simulink library "jud"  (Simulink 8.2)
settings: Solver=ode45  StartTime=0.0  StopTime=10.0  RelTol=1e-3
undefined symbols (not defined in the file or in its folder): ENUM_EPSADASABREASON_GEAR_POSITION_ERROR, ENUM_EPSADASABREASON_THERMAL_ERROR, ENUM_EPSADASABREASON_VEHICLE_SPEED_ERROR, ENUM_EPSLFCSTATUS_NOTAVAIL_PERM, ENUM_EPSLFCSTATUS_NOTAVAIL_TEMP, ENUM_EPSLFCSTATUS_OFF, ENUM_EPSLFCSTATUS_READY, ENUM_EPSLFCSTATUS_TRANSITION, ENUM_EPSLKASTATUS_NOTAVAIL_PERM, ENUM_EPSLKASTATUS_NOTAVAIL_TEMP, ENUM_EPSLKASTATUS_OFF, ENUM_EPSLKASTATUS_READY, ENUM_HMISTATE_ACTIVE, ENUM_KEYSWITCH_ON, ENUM_LFCSTATE_AUTOSTEERING, ENUM_LFCSTATE_STANDBY, ENUM_SENSORSTATE_NORMAL, FALSE, KAPP_VehicleWidth_m, KJUD_EPSLimition_kph, KJUD_EPSLimitionHysis_kph, KJUD_LFC4StandbyDelay_s, KJUD_SoftenTimerThr_s, TRUE, VJUD_LFCOffCount4LKAStandby_s, VJUD_LKAReActingDelay_s, VJUD_TLCTriggerReActingDelay_s
libraries: hcu_lib x12, simulink x10, jcc x1, jcw x1, jeb x1
(part 2 of 3)

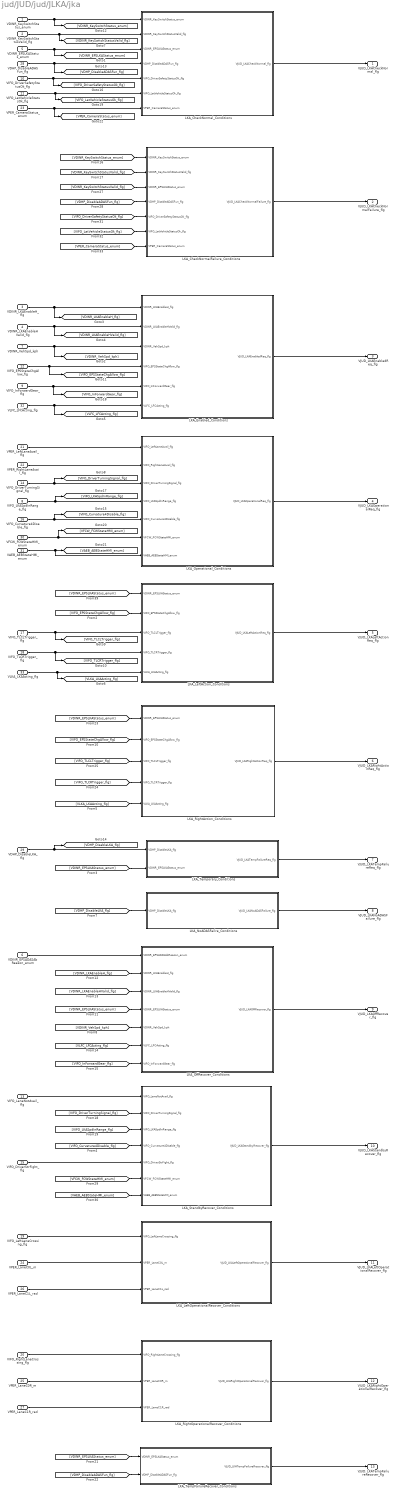
== system jud/JUD/jud/JLKA/jka ==
  VDINR_KeySwitchStatus_enum : Inport
  VDINR_KeySwitchStatusValid_flg : Inport  Port=2
  VDINR_LKAEnableH_flg : Inport  Port=3
  VDINR_LKAEnableHValid_flg : Inport  Port=4
  VDINR_EPSLKAStatus_enum : Inport  Port=5
  VDINR_EPSADASAbReason_enum : Inport  Port=6
  VDINR_VehSpd_kph : Inport  Port=7
  "VIFO_LKASpdInRange_flg " : Inport  Port=8
  VIFO_InForwardGear_flg : Inport  Port=9
  VIFO_DriverSafetyStatusOk_flg : Inport  Port=10
  VIFO_LatVehicleStatusOk_flg : Inport  Port=11
  VIFO_EPSStateChgAllow_flg : Inport  Port=12
  VIFO_LaneNotAvail_flg : Inport  Port=13
  VIFO_DriverTurningSignal_flg : Inport  Port=14
  VIFO_DriverStrFight_flg : Inport  Port=15
  VIFO_Curvature4Disable_flg : Inport  Port=16
  VIFO_TLCLTrigger_flg : Inport  Port=17
  VIFO_TLCRTrigger_flg : Inport  Port=18
  VIFO_LeftLaneCrossing_flg : Inport  Port=19
  VIFO_RightLaneCrossing_flg : Inport  Port=20
  VPER_LeftLaneAvail_flg : Inport  Port=21
  VPER_RightLaneAvail_flg : Inport  Port=22
  VPER_CameraStatus_enum : Inport  Port=23
  VPER_LaneC0L_m : Inport  Port=24
  VPER_LaneC0R_m : Inport  Port=25
  VPER_LaneC1L_rad : Inport  Port=26
  VPER_LaneC1R_rad : Inport  Port=27
  VDHP_DisableADASFun_flg : Inport  Port=28
  VDHP_DisableLKA_flg : Inport  Port=29
  VFCW_FCWStateHMI_enum : Inport  Port=30
  VAEB_AEBStateHMI_enum : Inport  Port=31
  VLFC_LFCActing_flg : Inport  Port=32
  VLKA_LKAActing_flg : Inport  Port=33
  LKA_CheckNormalFailure_Conditions : Subsystem
  LKA_CheckNormal_Conditions : Subsystem
  LKA_Enabled_Conditions : Subsystem
  LKA_LeftAction_Conditions : Subsystem
  LKA_LeftOperationalRecover_Conditions : Subsystem
  LKA_NoADASFailre_Conditions : Subsystem
  LKA_OffRecover_Conditions : Subsystem
  LKA_Operational_Conditions : Subsystem
  LKA_RightAction_Conditions : Subsystem
  LKA_RightOperationalRecover_Conditions : Subsystem
  LKA_StandbyRecover_Conditions : Subsystem
  LKA_TempFailureRecover_Conditions : Subsystem
  LKA_Temporary_Conditions : Subsystem
  VJUD_LKACheckNormal_flg : Outport
  VJUD_LKACheckNormalFailure_flg : Outport  Port=2
  VJUD_LKAEnabledReq_flg : Outport  Port=3
  VJUD_LKAOperationalReq_flg : Outport  Port=4
  VJUD_LKALeftActionReq_flg : Outport  Port=5
  VJUD_LKARightActionReq_flg : Outport  Port=6
  VJUD_LKATempFailureReq_flg : Outport  Port=7
  VJUD_LKANoADASFailure_flg : Outport  Port=8
  VJUD_LKAOffRecover_flg : Outport  Port=9
  VJUD_LKAStandbyRecover_flg : Outport  Port=10
  VJUD_LKALeftOperationalRecover_flg : Outport  Port=11
  VJUD_LKARightOperationalRecover_flg : Outport  Port=12
  VJUD_LKATempFailureRecover_flg : Outport  Port=13
  wires:
  LKA_CheckNormal_Conditions/1(VJUD_LKACheckNormal_flg) -> VJUD_LKACheckNormal_flg/1
  VDINR_KeySwitchStatusValid_flg/1 -> [VDINR_KeySwitchStatusValid_flg], LKA_CheckNormal_Conditions/2(VDINR_KeySwitchStatusValid_flg)
  LKA_Operational_Conditions/1(VJUD_LKAOperationalReq_flg) -> VJUD_LKAOperationalReq_flg/1
  VPER_LeftLaneAvail_flg/1 -> LKA_Operational_Conditions/1(VIFO_LeftLaneAvail_flg)
  VPER_RightLaneAvail_flg/1 -> LKA_Operational_Conditions/2(VIFO_RightLaneAvail_flg)
  VIFO_TLCLTrigger_flg/1 -> [VIFO_TLCLTrigger_flg], LKA_LeftAction_Conditions/3(VIFO_TLCLTrigger_flg)
  LKA_LeftAction_Conditions/1(VJUD_LKALeftActionReq_flg) -> VJUD_LKALeftActionReq_flg/1
  VIFO_DriverSafetyStatusOk_flg/1 -> [VIFO_DriverSafetyStatusOk_flg], LKA_CheckNormal_Conditions/5(VIFO_DriverSafetyStatusOk_flg)
  VDINR_LKAEnableH_flg/1 -> [VDINR_LKAEnableH_flg], LKA_Enabled_Conditions/1(VDINR_LKAEnableH_flg)
  VDINR_LKAEnableHValid_flg/1 -> [VDINR_LKAEnableHValid_flg], LKA_Enabled_Conditions/2(VDINR_LKAEnableHValid_flg)
  LKA_Enabled_Conditions/1(VJUD_LKAEnabledReq_flg) -> VJUD_LKAEnabledReq_flg/1
  VDHP_DisableADASFun_flg/1 -> [VDHP_DisableADASFun_flg], LKA_CheckNormal_Conditions/4(VDHP_DisableADASFun_flg)
  VIFO_EPSStateChgAllow_flg/1 -> [VIFO_EPSStateChgAllow_flg], LKA_Enabled_Conditions/4(VIFO_EPSStateChgAllow_flg)
  VDINR_EPSLKAStatus_enum/1 -> LKA_CheckNormal_Conditions/3(VDINR_EPSLKAStatus_enum), [VDINR_EPSLKAStatus_enum]
  [VDINR_EPSLKAStatus_enum] -> LKA_LeftAction_Conditions/1(VDINR_EPSLKAStatus_enum)
  VIFO_DriverTurningSignal_flg/1 -> [VIFO_DriverTurningSignal_flg], LKA_Operational_Conditions/3(VIFO_DriverTurningSignal_flg)
  VDINR_VehSpd_kph/1 -> [VDINR_VehSpd_kph], LKA_Enabled_Conditions/3(VDINR_VehSpd_kph)
  "VIFO_LKASpdInRange_flg "/1 -> [VIFO_LKASpdInRange_flg], LKA_Operational_Conditions/4(VIFO_LKASpdInRange_flg)
  [VIFO_EPSStateChgAllow_flg] -> LKA_LeftAction_Conditions/2(VIFO_EPSStateChgAllow_flg)
  LKA_Temporary_Conditions/1(VJUD_LKATempFailureReq_flg) -> VJUD_LKATempFailureReq_flg/1
  [VDINR_EPSLKAStatus_enum] -> LKA_Temporary_Conditions/2(VDINR_EPSLKAStatus_enum)
  LKA_NoADASFailre_Conditions/1(VJUD_LKANoADASFailure_flg) -> VJUD_LKANoADASFailure_flg/1
  [VDHP_DisableLKA_flg] -> LKA_NoADASFailre_Conditions/1(VDHP_DisableLKA_flg)
  LKA_OffRecover_Conditions/1(VJUD_LKAOffRecover_flg) -> VJUD_LKAOffRecover_flg/1
  VLFC_LFCActing_flg/1 -> [VLFC_LFCActing_flg], LKA_Enabled_Conditions/6(VLFC_LFCActing_flg)
  [VDINR_VehSpd_kph] -> LKA_OffRecover_Conditions/5(VDINR_VehSpd_kph)
  [VDINR_EPSLKAStatus_enum] -> LKA_OffRecover_Conditions/4(VDINR_EPSLKAStatus_enum)
  VDINR_EPSADASAbReason_enum/1 -> LKA_OffRecover_Conditions/1(VDINR_EPSADASAbReason_enum)
  [VDINR_LKAEnableH_flg] -> LKA_OffRecover_Conditions/2(VDINR_LKAEnableH_flg)
  [VDINR_LKAEnableHValid_flg] -> LKA_OffRecover_Conditions/3(VDINR_LKAEnableHValid_flg)
  [VLFC_LFCActing_flg] -> LKA_OffRecover_Conditions/6(VLFC_LFCActing_flg)
  LKA_StandbyRecover_Conditions/1(VJUD_LKAStandbyRecover_flg) -> VJUD_LKAStandbyRecover_flg/1
  [VIFO_LKASpdInRange_flg] -> LKA_StandbyRecover_Conditions/3(VIFO_LKASpdInRange_flg)
  LKA_LeftOperationalRecover_Conditions/1(VJUD_LKALeftOperationalRecover_flg) -> VJUD_LKALeftOperationalRecover_flg/1
  LKA_TempFailureRecover_Conditions/1(VJUD_LKATempFailureRecover_flg) -> VJUD_LKATempFailureRecover_flg/1
  [VDINR_EPSLKAStatus_enum] -> LKA_TempFailureRecover_Conditions/1(VDINR_EPSLKAStatus_enum)
  [VDHP_DisableADASFun_flg] -> LKA_TempFailureRecover_Conditions/2(VDHP_DisableADASFun_flg)
  VIFO_Curvature4Disable_flg/1 -> [VIFO_Curvature4Disable_flg], LKA_Operational_Conditions/5(VIFO_Curvature4Disable_flg)
  VDHP_DisableLKA_flg/1 -> LKA_Temporary_Conditions/1(VDHP_DisableLKA_flg), [VDHP_DisableLKA_flg]
  [VIFO_Curvature4Disable_flg] -> LKA_StandbyRecover_Conditions/4(VIFO_Curvature4Disable_flg)
  [VIFO_EPSStateChgAllow_flg] -> LKA_RightAction_Conditions/2(VIFO_EPSStateChgAllow_flg)
  [VDINR_EPSLKAStatus_enum] -> LKA_RightAction_Conditions/1(VDINR_EPSLKAStatus_enum)
  LKA_RightAction_Conditions/1(VJUD_LKARightActionReq_flg) -> VJUD_LKARightActionReq_flg/1
  VIFO_TLCRTrigger_flg/1 -> [VIFO_TLCRTrigger_flg], LKA_LeftAction_Conditions/4(VIFO_TLCRTrigger_flg)
  [VIFO_TLCRTrigger_flg] -> LKA_RightAction_Conditions/4(VIFO_TLCRTrigger_flg)
  [VIFO_TLCLTrigger_flg] -> LKA_RightAction_Conditions/3(VIFO_TLCLTrigger_flg)
  VIFO_LatVehicleStatusOk_flg/1 -> [VIFO_LatVehicleStatusOk_flg], LKA_CheckNormal_Conditions/6(VIFO_LatVehicleStatusOk_flg)
  VPER_CameraStatus_enum/1 -> [VPER_CameraStatus_enum], LKA_CheckNormal_Conditions/7(VPER_CameraStatus_enum)
  VIFO_InForwardGear_flg/1 -> LKA_Enabled_Conditions/5(VIFO_InForwardGear_flg), [VIFO_InForwardGear_flg]
  [VIFO_InForwardGear_flg] -> LKA_OffRecover_Conditions/7(VIFO_InForwardGear_flg)
  [VIFO_DriverTurningSignal_flg] -> LKA_StandbyRecover_Conditions/2(VIFO_DriverTurningSignal_flg)
  VIFO_LaneNotAvail_flg/1 -> LKA_StandbyRecover_Conditions/1(VIFO_LaneNotAvail_flg)
  VIFO_DriverStrFight_flg/1 -> LKA_StandbyRecover_Conditions/5(VIFO_DriverStrFight_flg)
  VFCW_FCWStateHMI_enum/1 -> [VFCW_FCWStateHMI_enum], LKA_Operational_Conditions/6(VFCW_FCWStateHMI_enum)
  VAEB_AEBStateHMI_enum/1 -> LKA_Operational_Conditions/7(VAEB_AEBStateHMI_enum), [VAEB_AEBStateHMI_enum]
  LKA_RightOperationalRecover_Conditions/1(VJUD_LKARightOperationalRecover_flg) -> VJUD_LKARightOperationalRecover_flg/1
  VPER_LaneC1L_rad/1 -> LKA_LeftOperationalRecover_Conditions/3(VPER_LaneC1L_rad)
  VPER_LaneC1R_rad/1 -> LKA_RightOperationalRecover_Conditions/3(VPER_LaneC1R_rad)
  [VFCW_FCWStateHMI_enum] -> LKA_StandbyRecover_Conditions/6(VFCW_FCWStateHMI_enum)
  [VAEB_AEBStateHMI_enum] -> LKA_StandbyRecover_Conditions/7(VAEB_AEBStateHMI_enum)
  VIFO_LeftLaneCrossing_flg/1 -> LKA_LeftOperationalRecover_Conditions/1(VIFO_LeftLaneCrossing_flg)
  VIFO_RightLaneCrossing_flg/1 -> LKA_RightOperationalRecover_Conditions/1(VIFO_RightLaneCrossing_flg)
  VPER_LaneC0L_m/1 -> LKA_LeftOperationalRecover_Conditions/2(VPER_LaneC0L_m)
  VPER_LaneC0R_m/1 -> LKA_RightOperationalRecover_Conditions/2(VPER_LaneC0R_m)
  VLKA_LKAActing_flg/1 -> [VLKA_LKAActing_flg], LKA_LeftAction_Conditions/5(VLKA_LKAActing_flg)
  [VLKA_LKAActing_flg] -> LKA_RightAction_Conditions/5(VLKA_LKAActing_flg)
  VDINR_KeySwitchStatus_enum/1 -> [VDINR_KeySwitchStatus_enum], LKA_CheckNormal_Conditions/1(VDINR_KeySwitchStatus_enum)
  [VDINR_KeySwitchStatus_enum] -> LKA_CheckNormalFailure_Conditions/1(VDINR_KeySwitchStatus_enum)
  [VDINR_KeySwitchStatusValid_flg] -> LKA_CheckNormalFailure_Conditions/2(VDINR_KeySwitchStatusValid_flg)
  [VDINR_KeySwitchStatusValid_flg] -> LKA_CheckNormalFailure_Conditions/3(VDINR_EPSLKAStatus_enum)
  [VDHP_DisableADASFun_flg] -> LKA_CheckNormalFailure_Conditions/4(VDHP_DisableADASFun_flg)
  [VIFO_DriverSafetyStatusOk_flg] -> LKA_CheckNormalFailure_Conditions/5(VIFO_DriverSafetyStatusOk_flg)
  [VIFO_LatVehicleStatusOk_flg] -> LKA_CheckNormalFailure_Conditions/6(VIFO_LatVehicleStatusOk_flg)
  [VPER_CameraStatus_enum] -> LKA_CheckNormalFailure_Conditions/7(VPER_CameraStatus_enum)
  LKA_CheckNormalFailure_Conditions/1(VJUD_LKACheckNormalFailure_flg) -> VJUD_LKACheckNormalFailure_flg/1

== system jud/JUD/jud/JLCA/jca/LCA_CheckNormal_Conditions ==
  VDINR_KeySwitchStatus_enum : Inport
  VDINR_KeySwitchStatusValid_flg : Inport  Port=2
  VDHP_DisableADASFun_flg : Inport  Port=3
  VIFO_DriverSafetyStatusOk_flg : Inport  Port=4
  VIFO_LatVehicleStatusOk_flg : Inport  Port=5
  VPER_CameraStatus_enum : Inport  Port=6
  Constant : Constant  Value=ENUM_KEYSWITCH_ON
  Constant2 : Constant  Value=ENUM_SENSORSTATE_NORMAL
  Logical Operator : Logic  Inputs=6  AllPortsSameDT=off  OutDataTypeStr=boolean
  Logical Operator1 : Logic  Operator=NOT  AllPortsSameDT=off  OutDataTypeStr=boolean
  Relational Operator : RelationalOperator  Operator===  OutDataTypeStr=boolean
  Relational Operator2 : RelationalOperator  Operator===  OutDataTypeStr=boolean
  VJUD_LCACheckNormal_flg : Outport
  wires:
  Logical Operator/1 -> VJUD_LCACheckNormal_flg/1  "VJUD_LCACheckNormal_flg"
  VDINR_KeySwitchStatus_enum/1 -> Relational Operator/1
  Constant/1 -> Relational Operator/2
  Relational Operator/1 -> Logical Operator/1
  VDINR_KeySwitchStatusValid_flg/1 -> Logical Operator/2
  VIFO_DriverSafetyStatusOk_flg/1 -> Logical Operator/3
  VDHP_DisableADASFun_flg/1 -> Logical Operator1/1
  Relational Operator2/1 -> Logical Operator/5
  VPER_CameraStatus_enum/1 -> Relational Operator2/1
  Constant2/1 -> Relational Operator2/2
  VIFO_LatVehicleStatusOk_flg/1 -> Logical Operator/4
  Logical Operator1/1 -> Logical Operator/6

== system jud/JUD/jud/JLCA/jca/LCA_Enabled_Conditions ==
  VDINR_LCAEnableH_flg : Inport
  VDINR_LCAEnableHValid_flg : Inport  Port=2
  VDINR_VehSpd_kph : Inport  Port=3
  VIFO_InForwardGear_flg : Inport  Port=4
  VDHP_DisableADASFun_flg : Inport  Port=5
  Constant1 : Constant  Value=KJUD_EPSLimition_kph
  Logical Operator : Logic  Inputs=5  AllPortsSameDT=off  OutDataTypeStr=boolean
  Logical Operator1 : Logic  Operator=NOT  AllPortsSameDT=off  OutDataTypeStr=boolean
  Relational Operator7 : RelationalOperator  OutDataTypeStr=boolean
  VJUD_LCAEnabledReq_flg : Outport
  wires:
  VDINR_LCAEnableH_flg/1 -> Logical Operator/1
  Logical Operator/1 -> VJUD_LCAEnabledReq_flg/1  "VJUD_LCAEnabledReq_flg"
  VDINR_LCAEnableHValid_flg/1 -> Logical Operator/2
  VDHP_DisableADASFun_flg/1 -> Logical Operator1/1
  VDINR_VehSpd_kph/1 -> Relational Operator7/1
  Constant1/1 -> Relational Operator7/2
  Relational Operator7/1 -> Logical Operator/3
  VIFO_InForwardGear_flg/1 -> Logical Operator/4
  Logical Operator1/1 -> Logical Operator/5

== system jud/JUD/jud/JLCA/jca/LCA_LeftAction_Conditions ==
  VIFO_DriverTurningSignalSwL_flg : Inport
  Constant : Constant  Value=2
  Detect Decrease : simulink/Logic and Bit Operations/Detect Decrease  vinit=0.0  InputProcessing=Inherited  OutDataTypeStr=boolean
  Detect Increase : simulink/Logic and Bit Operations/Detect Increase  vinit=0.0  InputProcessing=Inherited  OutDataTypeStr=boolean
  Detect Increase1 : simulink/Logic and Bit Operations/Detect Increase  vinit=0.0  InputProcessing=Inherited  OutDataTypeStr=boolean
  Relational Operator : RelationalOperator  OutDataTypeStr=boolean
  SR-Latch : hcu_lib/SR-Latch  SystemSampleTime=-1
  Timer : hcu_lib/Timer  SystemSampleTime=-1
  VJUD_LCALeftActionReq_flg : Outport
  wires:
  Constant/1 -> Relational Operator/2
  VIFO_DriverTurningSignalSwL_flg/1 -> Detect Decrease/1, Detect Increase/1
  Detect Increase/1 -> SR-Latch/1
  SR-Latch/1 -> Timer/Enable
  Timer/1 -> Relational Operator/1
  Relational Operator/1 -> Detect Increase1/1
  Detect Increase1/1 -> VJUD_LCALeftActionReq_flg/1  "VJUD_LCALeftActionReq_flg"
  Detect Decrease/1 -> SR-Latch/2

== system jud/JUD/jud/JLCA/jca/LCA_LeftOperationalRecover_Conditions ==
  VIFO_DriverTurningSignalSwL_flg : Inport
  VDINR_LaneCrossL_flg : Inport  Port=2
  Constant : Constant  Value=FALSE
  Logical Operator : Logic  Operator=OR  AllPortsSameDT=off  OutDataTypeStr=boolean
  Relational Operator : RelationalOperator  Operator===  OutDataTypeStr=boolean
  VJUD_LCALeftOperationalRecover_flg : Outport
  wires:
  Logical Operator/1 -> VJUD_LCALeftOperationalRecover_flg/1  "VJUD_LCALeftOperationalRecover_flg"
  VIFO_DriverTurningSignalSwL_flg/1 -> Relational Operator/1
  Constant/1 -> Relational Operator/2
  VDINR_LaneCrossL_flg/1 -> Logical Operator/2
  Relational Operator/1 -> Logical Operator/1

== system jud/JUD/jud/JLCA/jca/LCA_NoADASFailre_Conditions ==
  VDHP_DisableLFC_flg : Inport
  Logical Operator : Logic  Operator=NOT  AllPortsSameDT=off  OutDataTypeStr=boolean
  VJUD_LCANoADASFailure_flg : Outport
  wires:
  VDHP_DisableLFC_flg/1 -> Logical Operator/1
  Logical Operator/1 -> VJUD_LCANoADASFailure_flg/1  "VJUD_LCANoADASFailure_flg"

== system jud/JUD/jud/JLCA/jca/LCA_OffRecover_Conditions ==
  VDINR_LKAEnableH_flg : Inport
  VDINR_LKAEnableHValid_flg : Inport  Port=2
  VDINR_VehSpd_kph : Inport  Port=3
  VDHP_DisableADASFun_flg : Inport  Port=4
  VIFO_InForwardGear_flg : Inport  Port=5
  Add : Sum  Inputs=+-
  Constant14 : Constant  Value=KJUD_EPSLimition_kph
  Constant15 : Constant  Value=KJUD_EPSLimitionHysis_kph
  Logical Operator : Logic  Operator=OR  Inputs=5  AllPortsSameDT=off  OutDataTypeStr=boolean
  Logical Operator1 : Logic  Operator=NOT  AllPortsSameDT=off  OutDataTypeStr=boolean
  Logical Operator2 : Logic  Operator=NOT  AllPortsSameDT=off  OutDataTypeStr=boolean
  Logical Operator6 : Logic  Operator=NOT  AllPortsSameDT=off  OutDataTypeStr=boolean
  Relational Operator13 : RelationalOperator  Operator=<=  OutDataTypeStr=boolean
  VJUD_LCAOffRecover_flg : Outport
  wires:
  Logical Operator/1 -> VJUD_LCAOffRecover_flg/1  "VJUD_LCAOffRecover_flg"
  VDINR_LKAEnableH_flg/1 -> Logical Operator1/1
  VDINR_LKAEnableHValid_flg/1 -> Logical Operator2/1
  VDINR_VehSpd_kph/1 -> Relational Operator13/1
  Constant14/1 -> Add/1
  Constant15/1 -> Add/2
  Add/1 -> Relational Operator13/2
  Logical Operator1/1 -> Logical Operator/1
  Logical Operator2/1 -> Logical Operator/2
  Relational Operator13/1 -> Logical Operator/4
  Logical Operator6/1 -> Logical Operator/5
  VIFO_InForwardGear_flg/1 -> Logical Operator6/1
  VDHP_DisableADASFun_flg/1 -> Logical Operator/3

== system jud/JUD/jud/JLCA/jca/LCA_Operational_Conditions ==
  VFCW_FCWStateHMI_enum : Inport
  VAEB_AEBStateHMI_enum : Inport  Port=2
  VLFC_LFCState_enum : Inport  Port=3
  VLFC_LFCActing_flg : Inport  Port=4
  Constant1 : Constant  Value=ENUM_HMISTATE_ACTIVE
  Constant2 : Constant  Value=ENUM_HMISTATE_ACTIVE
  Constant3 : Constant  Value=ENUM_LFCSTATE_AUTOSTEERING
  Logical Operator : Logic  Inputs=4  AllPortsSameDT=off  OutDataTypeStr=boolean
  Relational Operator1 : RelationalOperator  Operator===  OutDataTypeStr=boolean
  Relational Operator2 : RelationalOperator  Operator=~=  OutDataTypeStr=boolean
  Relational Operator3 : RelationalOperator  Operator=~=  OutDataTypeStr=boolean
  VJUD_LCAOperationalReq_flg : Outport
  wires:
  Logical Operator/1 -> VJUD_LCAOperationalReq_flg/1  "VJUD_LCAOperationalReq_flg"
  VFCW_FCWStateHMI_enum/1 -> Relational Operator2/1
  VAEB_AEBStateHMI_enum/1 -> Relational Operator3/1
  Constant1/1 -> Relational Operator2/2
  Constant2/1 -> Relational Operator3/2
  VLFC_LFCState_enum/1 -> Relational Operator1/1
  Constant3/1 -> Relational Operator1/2
  Relational Operator2/1 -> Logical Operator/1
  Relational Operator3/1 -> Logical Operator/2
  Relational Operator1/1 -> Logical Operator/3
  VLFC_LFCActing_flg/1 -> Logical Operator/4

== system jud/JUD/jud/JLCA/jca/LCA_RightAction_Conditions ==
  VIFO_DriverTurningSignalSwR_flg : Inport
  Constant1 : Constant  Value=2
  Detect Decrease : simulink/Logic and Bit Operations/Detect Decrease  vinit=0.0  InputProcessing=Inherited  OutDataTypeStr=boolean
  Detect Increase : simulink/Logic and Bit Operations/Detect Increase  vinit=0.0  InputProcessing=Inherited  OutDataTypeStr=boolean
  Detect Increase1 : simulink/Logic and Bit Operations/Detect Increase  vinit=0.0  InputProcessing=Inherited  OutDataTypeStr=boolean
  Relational Operator1 : RelationalOperator  OutDataTypeStr=boolean
  SR-Latch : hcu_lib/SR-Latch  SystemSampleTime=-1
  Timer : hcu_lib/Timer  SystemSampleTime=-1
  VJUD_LCARightActionReq_flg : Outport
  wires:
  Constant1/1 -> Relational Operator1/2
  VIFO_DriverTurningSignalSwR_flg/1 -> Detect Decrease/1, Detect Increase/1
  Detect Increase/1 -> SR-Latch/1
  SR-Latch/1 -> Timer/Enable
  Timer/1 -> Relational Operator1/1
  Relational Operator1/1 -> Detect Increase1/1
  Detect Decrease/1 -> SR-Latch/2
  Detect Increase1/1 -> VJUD_LCARightActionReq_flg/1  "VJUD_LCARightActionReq_flg"

== system jud/JUD/jud/JLCA/jca/LCA_RightOperationalRecover_Conditions ==
  VIFO_DriverTurningSignalSwR_flg : Inport
  VDINR_LaneCrossR_flg : Inport  Port=2
  Constant : Constant  Value=FALSE
  Logical Operator : Logic  Operator=OR  AllPortsSameDT=off  OutDataTypeStr=boolean
  Relational Operator2 : RelationalOperator  Operator===  OutDataTypeStr=boolean
  VJUD_LCARightOperationalRecover_flg : Outport
  wires:
  VIFO_DriverTurningSignalSwR_flg/1 -> Relational Operator2/1
  Logical Operator/1 -> VJUD_LCARightOperationalRecover_flg/1  "VJUD_LCARightOperationalRecover_flg"
  Constant/1 -> Relational Operator2/2
  Relational Operator2/1 -> Logical Operator/1
  VDINR_LaneCrossR_flg/1 -> Logical Operator/2

== system jud/JUD/jud/JLCA/jca/LCA_StandbyRecover_Conditions ==
  VFCW_FCWStateHMI_enum : Inport
  VAEB_AEBStateHMI_enum : Inport  Port=2
  VLFC_LFCActing_flg : Inport  Port=3
  Constant1 : Constant  Value=ENUM_HMISTATE_ACTIVE
  Constant2 : Constant  Value=ENUM_HMISTATE_ACTIVE
  Logical Operator : Logic  Operator=OR  Inputs=3  AllPortsSameDT=off  OutDataTypeStr=boolean
  Logical Operator1 : Logic  Operator=NOT  AllPortsSameDT=off  OutDataTypeStr=boolean
  Relational Operator2 : RelationalOperator  Operator===  OutDataTypeStr=boolean
  Relational Operator3 : RelationalOperator  Operator===  OutDataTypeStr=boolean
  VJUD_LCAStandbyRecover_flg : Outport
  wires:
  Logical Operator/1 -> VJUD_LCAStandbyRecover_flg/1  "VJUD_LCAStandbyRecover_flg"
  VFCW_FCWStateHMI_enum/1 -> Relational Operator2/1
  VAEB_AEBStateHMI_enum/1 -> Relational Operator3/1
  Constant1/1 -> Relational Operator2/2
  Constant2/1 -> Relational Operator3/2
  Relational Operator2/1 -> Logical Operator/1
  Relational Operator3/1 -> Logical Operator/2
  VLFC_LFCActing_flg/1 -> Logical Operator1/1
  Logical Operator1/1 -> Logical Operator/3

== system jud/JUD/jud/JLCA/jca/LCA_TempFailureRecover_Conditions ==
  VDHP_DisableADASFun_flg : Inport
  VDINR_EPSLFCStatus_enum : Inport  Port=2
  Constant : Constant  Value=ENUM_EPSLFCSTATUS_OFF
  Constant1 : Constant  Value=ENUM_EPSLFCSTATUS_NOTAVAIL_PERM
  Logical Operator : Logic  Operator=OR  Inputs=3  AllPortsSameDT=off  OutDataTypeStr=boolean
  Relational Operator : RelationalOperator  Operator===  OutDataTypeStr=boolean
  Relational Operator1 : RelationalOperator  Operator===  OutDataTypeStr=boolean
  VJUD_LCATempFailureRecover_flg : Outport
  wires:
  VDHP_DisableADASFun_flg/1 -> Logical Operator/3
  Logical Operator/1 -> VJUD_LCATempFailureRecover_flg/1  "VJUD_LCATempFailureRecover_flg"
  Relational Operator/1 -> Logical Operator/1
  Constant/1 -> Relational Operator/2
  Relational Operator1/1 -> Logical Operator/2
  VDINR_EPSLFCStatus_enum/1 -> Relational Operator1/1, Relational Operator/1
  Constant1/1 -> Relational Operator1/2

== system jud/JUD/jud/JLCA/jca/LCA_Temporary_Conditions ==
  VDHP_DisableLFC_flg : Inport
  VDINR_EPSLFCStatus_enum : Inport  Port=2
  Constant : Constant  Value=ENUM_EPSLFCSTATUS_NOTAVAIL_TEMP
  Logical Operator1 : Logic  Operator=OR  AllPortsSameDT=off  OutDataTypeStr=boolean
  Relational Operator : RelationalOperator  Operator===  OutDataTypeStr=boolean
  VJUD_LCATempFailureReq_flg : Outport
  wires:
  VDHP_DisableLFC_flg/1 -> Logical Operator1/1
  Logical Operator1/1 -> VJUD_LCATempFailureReq_flg/1  "VJUD_LCATempFailureReq_flg"
  VDINR_EPSLFCStatus_enum/1 -> Relational Operator/1
  Constant/1 -> Relational Operator/2
  Relational Operator/1 -> Logical Operator1/2

== system jud/JUD/jud/JLFC/jfc/LFC_Action_Conditions ==
  VDINR_LFCOnVCU_flg : Inport
  VDINR_LFCOnVCUValid_flg : Inport  Port=2
  VDINR_EPSLFCStatus_enum : Inport  Port=3
  VIFO_EPSStateChgAllow_flg : Inport  Port=4
  Constant : Constant  Value=ENUM_EPSLFCSTATUS_READY
  Logical Operator : Logic  Inputs=4  AllPortsSameDT=off  OutDataTypeStr=boolean
  Relational Operator : RelationalOperator  Operator===  OutDataTypeStr=boolean
  VJUD_LFCActionReq_flg : Outport
  wires:
  Logical Operator/1 -> VJUD_LFCActionReq_flg/1  "VJUD_LFCActionReq_flg"
  VDINR_EPSLFCStatus_enum/1 -> Relational Operator/1
  Constant/1 -> Relational Operator/2
  VDINR_LFCOnVCU_flg/1 -> Logical Operator/1
  VDINR_LFCOnVCUValid_flg/1 -> Logical Operator/2
  Relational Operator/1 -> Logical Operator/3
  VIFO_EPSStateChgAllow_flg/1 -> Logical Operator/4

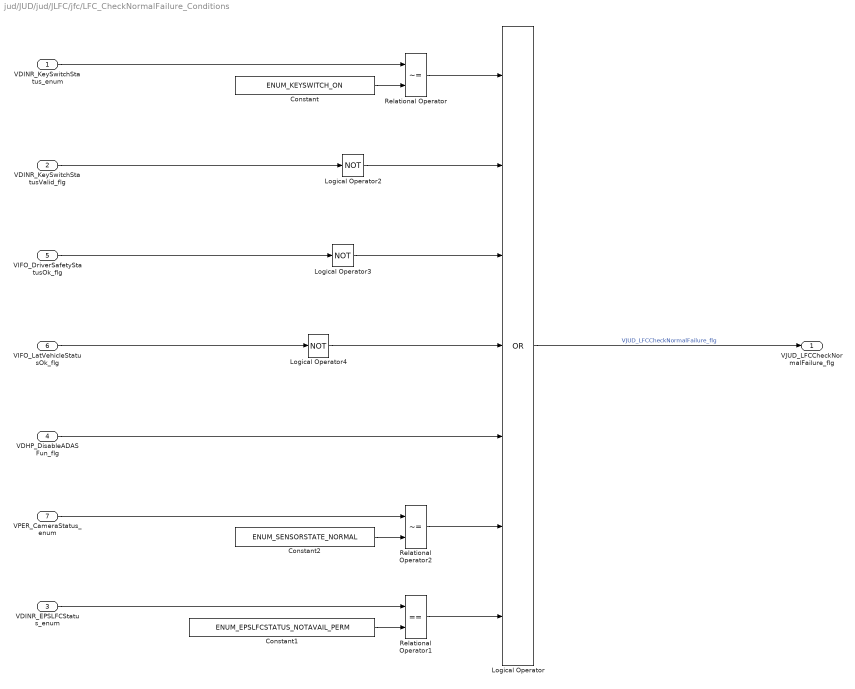
== system jud/JUD/jud/JLFC/jfc/LFC_CheckNormalFailure_Conditions ==
  VDINR_KeySwitchStatus_enum : Inport
  VDINR_KeySwitchStatusValid_flg : Inport  Port=2
  VDINR_EPSLFCStatus_enum : Inport  Port=3
  VDHP_DisableADASFun_flg : Inport  Port=4
  VIFO_DriverSafetyStatusOk_flg : Inport  Port=5
  VIFO_LatVehicleStatusOk_flg : Inport  Port=6
  VPER_CameraStatus_enum : Inport  Port=7
  Constant : Constant  Value=ENUM_KEYSWITCH_ON
  Constant1 : Constant  Value=ENUM_EPSLFCSTATUS_NOTAVAIL_PERM
  Constant2 : Constant  Value=ENUM_SENSORSTATE_NORMAL
  Logical Operator : Logic  Operator=OR  Inputs=7  AllPortsSameDT=off  OutDataTypeStr=boolean
  Logical Operator2 : Logic  Operator=NOT  AllPortsSameDT=off  OutDataTypeStr=boolean
  Logical Operator3 : Logic  Operator=NOT  AllPortsSameDT=off  OutDataTypeStr=boolean
  Logical Operator4 : Logic  Operator=NOT  AllPortsSameDT=off  OutDataTypeStr=boolean
  Relational Operator : RelationalOperator  Operator=~=  OutDataTypeStr=boolean
  Relational Operator1 : RelationalOperator  Operator===  OutDataTypeStr=boolean
  Relational Operator2 : RelationalOperator  Operator=~=  OutDataTypeStr=boolean
  VJUD_LFCCheckNormalFailure_flg : Outport
  wires:
  VDHP_DisableADASFun_flg/1 -> Logical Operator/5
  Constant2/1 -> Relational Operator2/2
  VPER_CameraStatus_enum/1 -> Relational Operator2/1
  VIFO_LatVehicleStatusOk_flg/1 -> Logical Operator4/1
  Constant1/1 -> Relational Operator1/2
  VDINR_EPSLFCStatus_enum/1 -> Relational Operator1/1
  VIFO_DriverSafetyStatusOk_flg/1 -> Logical Operator3/1
  VDINR_KeySwitchStatusValid_flg/1 -> Logical Operator2/1
  Relational Operator/1 -> Logical Operator/1
  Constant/1 -> Relational Operator/2
  VDINR_KeySwitchStatus_enum/1 -> Relational Operator/1
  Logical Operator/1 -> VJUD_LFCCheckNormalFailure_flg/1  "VJUD_LFCCheckNormalFailure_flg"
  Relational Operator2/1 -> Logical Operator/6
  Logical Operator2/1 -> Logical Operator/2
  Logical Operator3/1 -> Logical Operator/3
  Logical Operator4/1 -> Logical Operator/4
  Relational Operator1/1 -> Logical Operator/7

== system jud/JUD/jud/JLFC/jfc/LFC_CheckNormal_Conditions ==
  VDINR_KeySwitchStatus_enum : Inport
  VDINR_KeySwitchStatusValid_flg : Inport  Port=2
  VDINR_EPSLFCStatus_enum : Inport  Port=3
  VDHP_DisableADASFun_flg : Inport  Port=4
  VIFO_DriverSafetyStatusOk_flg : Inport  Port=5
  VIFO_LatVehicleStatusOk_flg : Inport  Port=6
  VPER_CameraStatus_enum : Inport  Port=7
  Constant : Constant  Value=ENUM_KEYSWITCH_ON
  Constant1 : Constant  Value=ENUM_EPSLFCSTATUS_OFF
  Constant2 : Constant  Value=ENUM_SENSORSTATE_NORMAL
  Logical Operator : Logic  Inputs=7  AllPortsSameDT=off  OutDataTypeStr=boolean
  Logical Operator1 : Logic  Operator=NOT  AllPortsSameDT=off  OutDataTypeStr=boolean
  Relational Operator : RelationalOperator  Operator===  OutDataTypeStr=boolean
  Relational Operator1 : RelationalOperator  Operator===  OutDataTypeStr=boolean
  Relational Operator2 : RelationalOperator  Operator===  OutDataTypeStr=boolean
  VJUD_LFCCheckNormal_flg : Outport
  wires:
  Logical Operator/1 -> VJUD_LFCCheckNormal_flg/1  "VJUD_LFCCheckNormal_flg"
  VDINR_KeySwitchStatus_enum/1 -> Relational Operator/1
  Constant/1 -> Relational Operator/2
  Relational Operator/1 -> Logical Operator/1
  VDINR_KeySwitchStatusValid_flg/1 -> Logical Operator/2
  VIFO_DriverSafetyStatusOk_flg/1 -> Logical Operator/3
  VDHP_DisableADASFun_flg/1 -> Logical Operator1/1
  VDINR_EPSLFCStatus_enum/1 -> Relational Operator1/1
  Constant1/1 -> Relational Operator1/2
  VIFO_LatVehicleStatusOk_flg/1 -> Logical Operator/4
  Relational Operator2/1 -> Logical Operator/5
  VPER_CameraStatus_enum/1 -> Relational Operator2/1
  Constant2/1 -> Relational Operator2/2
  Relational Operator1/1 -> Logical Operator/6
  Logical Operator1/1 -> Logical Operator/7

== system jud/JUD/jud/JLFC/jfc/LFC_Degraded_Conditions ==
  VIFO_LaneNotAvail_flg : Inport
  Logical Operator : Logic  Operator=OR  Inputs=1  AllPortsSameDT=off  OutDataTypeStr=boolean
  VJUD_LFCDegradedReq_flg : Outport
  wires:
  VIFO_LaneNotAvail_flg/1 -> Logical Operator/1
  Logical Operator/1 -> VJUD_LFCDegradedReq_flg/1  "VJUD_LFCDegradedReq_flg"

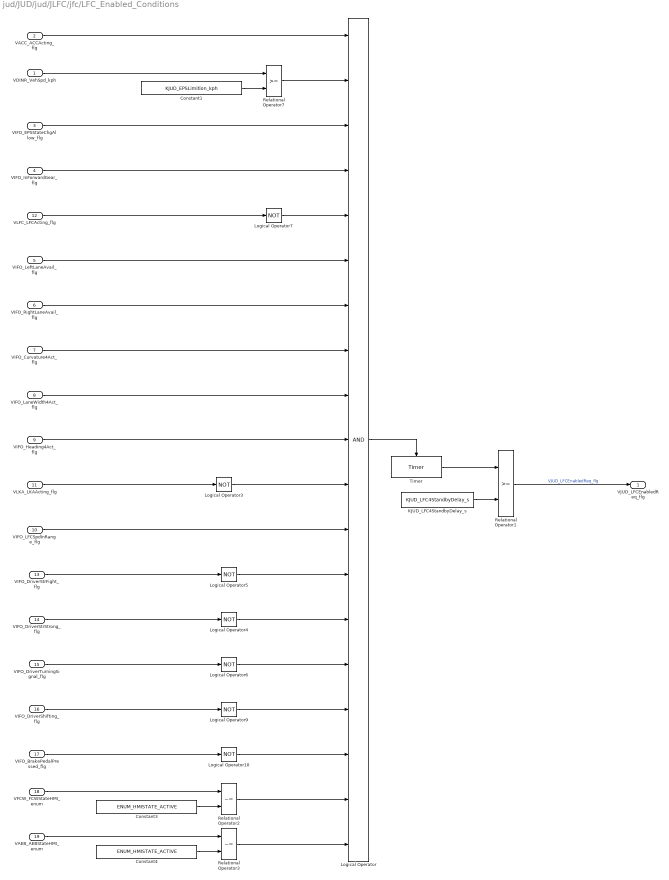
== system jud/JUD/jud/JLFC/jfc/LFC_Enabled_Conditions ==
  VDINR_VehSpd_kph : Inport
  VACC_ACCActing_flg : Inport  Port=2
  VIFO_EPSStateChgAllow_flg : Inport  Port=3
  "VIFO_InForwardGear_flg " : Inport  Port=4
  VIFO_LeftLaneAvail_flg : Inport  Port=5
  VIFO_RightLaneAvail_flg : Inport  Port=6
  VIFO_Curvature4Act_flg : Inport  Port=7
  VIFO_LaneWidth4Act_flg : Inport  Port=8
  VIFO_Heading4Act_flg : Inport  Port=9
  VIFO_LFCSpdInRange_flg : Inport  Port=10
  VLKA_LKAActing_flg : Inport  Port=11
  VLFC_LFCActing_flg : Inport  Port=12
  VIFO_DriverStrFight_flg : Inport  Port=13
  VIFO_DriverStrStrong_flg : Inport  Port=14
  VIFO_DriverTurningSignal_flg : Inport  Port=15
  VIFO_DriverShifting_flg : Inport  Port=16
  VIFO_BrakePedalPressed_flg : Inport  Port=17
  VFCW_FCWStateHMI_enum : Inport  Port=18
  VAEB_AEBStateHMI_enum : Inport  Port=19
  Constant1 : Constant  Value=KJUD_EPSLimition_kph
  Constant3 : Constant  Value=ENUM_HMISTATE_ACTIVE
  Constant4 : Constant  Value=ENUM_HMISTATE_ACTIVE
  KJUD_LFC4StandbyDelay_s : Constant  Value=KJUD_LFC4StandbyDelay_s  OutDataTypeStr=single
  Logical Operator : Logic  Inputs=19  AllPortsSameDT=off  OutDataTypeStr=boolean
  Logical Operator{3..7,9..10} (7 alike) : Logic  Operator=NOT  Inputs=1  AllPortsSameDT=off  OutDataTypeStr=boolean
  Relational Operator1 : RelationalOperator  OutDataTypeStr=boolean
  Relational Operator2 : RelationalOperator  Operator=~=  OutDataTypeStr=boolean
  Relational Operator3 : RelationalOperator  Operator=~=  OutDataTypeStr=boolean
  Relational Operator7 : RelationalOperator  OutDataTypeStr=boolean
  Timer : hcu_lib/Timer  SystemSampleTime=-1
  VJUD_LFCEnabledReq_flg : Outport
  wires:
  Logical Operator/1 -> Timer/Enable
  VDINR_VehSpd_kph/1 -> Relational Operator7/1
  Constant1/1 -> Relational Operator7/2
  VACC_ACCActing_flg/1 -> Logical Operator/1
  Relational Operator7/1 -> Logical Operator/2
  VLKA_LKAActing_flg/1 -> Logical Operator3/1
  VLFC_LFCActing_flg/1 -> Logical Operator7/1
  VIFO_DriverStrStrong_flg/1 -> Logical Operator4/1
  VFCW_FCWStateHMI_enum/1 -> Relational Operator2/1
  VAEB_AEBStateHMI_enum/1 -> Relational Operator3/1
  Constant3/1 -> Relational Operator2/2
  Constant4/1 -> Relational Operator3/2
  VIFO_DriverStrFight_flg/1 -> Logical Operator5/1
  VIFO_DriverTurningSignal_flg/1 -> Logical Operator6/1
  VIFO_DriverShifting_flg/1 -> Logical Operator9/1
  VIFO_BrakePedalPressed_flg/1 -> Logical Operator10/1
  Timer/1 -> Relational Operator1/1
  KJUD_LFC4StandbyDelay_s/1 -> Relational Operator1/2
  Relational Operator1/1 -> VJUD_LFCEnabledReq_flg/1  "VJUD_LFCEnabledReq_flg"
  "VIFO_InForwardGear_flg "/1 -> Logical Operator/4
  VIFO_EPSStateChgAllow_flg/1 -> Logical Operator/3
  Logical Operator7/1 -> Logical Operator/5
  VIFO_LaneWidth4Act_flg/1 -> Logical Operator/9
  VIFO_Curvature4Act_flg/1 -> Logical Operator/8
  VIFO_RightLaneAvail_flg/1 -> Logical Operator/7
  VIFO_LeftLaneAvail_flg/1 -> Logical Operator/6
  VIFO_Heading4Act_flg/1 -> Logical Operator/10
  Logical Operator3/1 -> Logical Operator/11
  VIFO_LFCSpdInRange_flg/1 -> Logical Operator/12
  Logical Operator5/1 -> Logical Operator/13
  Logical Operator4/1 -> Logical Operator/14
  Logical Operator6/1 -> Logical Operator/15
  Logical Operator10/1 -> Logical Operator/17
  Logical Operator9/1 -> Logical Operator/16
  Relational Operator2/1 -> Logical Operator/18
  Relational Operator3/1 -> Logical Operator/19

== system jud/JUD/jud/JLFC/jfc/LFC_NoADASFailre_Conditions ==
  VDHP_DisableLFC_flg : Inport
  Logical Operator2 : Logic  Operator=NOT  AllPortsSameDT=off  OutDataTypeStr=boolean
  VJUD_LFCNoADASFailure_flg : Outport
  wires:
  Logical Operator2/1 -> VJUD_LFCNoADASFailure_flg/1  "VJUD_LFCNoADASFailure_flg"
  VDHP_DisableLFC_flg/1 -> Logical Operator2/1

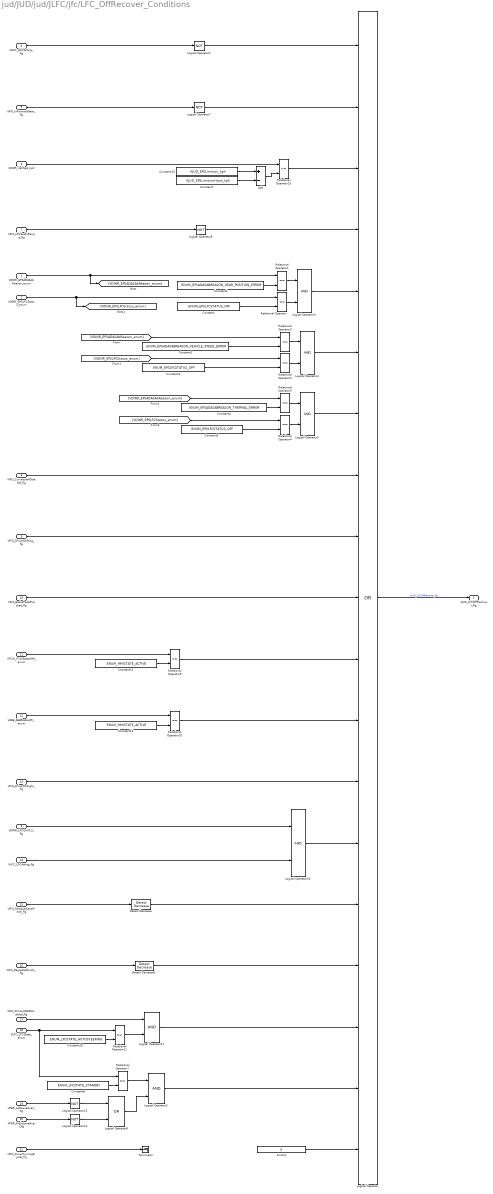
== system jud/JUD/jud/JLFC/jfc/LFC_OffRecover_Conditions ==
  VDINR_EPSADASAbReason_enum : Inport
  VDINR_EPSLFCStatus_enum : Inport  Port=2
  VDINR_VehSpd_kph : Inport  Port=3
  VACC_ACCActing_flg : Inport  Port=4
  VIFO_InForwardGear_flg : Inport  Port=5
  VIFO_Curvature4Disable_flg : Inport  Port=6
  VIFO_LFCSpdInRange_flg : Inport  Port=7
  VDINR_LFCOnVCU_flg : Inport  Port=8
  VIFO_DriverShifting_flg : Inport  Port=9
  VIFO_BrakePedalPressed_flg : Inport  Port=10
  VFCW_FCWStateHMI_enum : Inport  Port=11
  VAEB_AEBStateHMI_enum : Inport  Port=12
  VIFO_DriverStrFight_flg : Inport  Port=13
  VLFC_LFCActing_flg : Inport  Port=14
  VIFO_ResidualLaneFinish_flg : Inport  Port=15
  VIFO_DegradedFinish_flg : Inport  Port=16
  VIFO_DriverHOD4Disabled_flg : Inport  Port=17
  VLFC_LFCState_enum : Inport  Port=18
  VPER_LeftLaneAvail_flg : Inport  Port=19
  VPER_RightLaneAvail_flg : Inport  Port=20
  VIFO_DriverTurningSignal_flg : Inport  Port=21
  Add : Sum  Inputs=+-
  Constant : Constant  Value=ENUM_EPSLFCSTATUS_OFF
  Constant1 : Constant  Value=ENUM_EPSADASABREASON_GEAR_POSITION_ERROR
  Constant10 : Constant  Value=ENUM_LFCSTATE_AUTOSTEERING
  Constant12 : Constant  Value=ENUM_HMISTATE_ACTIVE
  Constant13 : Constant  Value=KJUD_EPSLimition_kph
  Constant14 : Constant  Value=ENUM_HMISTATE_ACTIVE
  Constant2 : Constant  Value=ENUM_EPSADASABREASON_VEHICLE_SPEED_ERROR
  Constant3 : Constant  Value=ENUM_EPSLFCSTATUS_OFF
  Constant4 : Constant  Value=ENUM_EPSADASABREASON_THERMAL_ERROR
  Constant5 : Constant  Value=ENUM_EPSLFCSTATUS_OFF
  Constant7 : Constant  Value=KJUD_EPSLimitionHysis_kph
  Constant8 : Constant  Value=ENUM_LFCSTATE_STANDBY
  Detect Decrease : simulink/Logic and Bit Operations/Detect Decrease  vinit=0.0  InputProcessing=Inherited  OutDataTypeStr=boolean
  Detect Decrease1 : simulink/Logic and Bit Operations/Detect Decrease  vinit=0.0  InputProcessing=Inherited  OutDataTypeStr=boolean
  ForLCA : Constant  Value=0  OutDataTypeStr=boolean
  Logical Operator : Logic  Operator=OR  Inputs=19  AllPortsSameDT=off  OutDataTypeStr=boolean
  Logical Operator{1,7..8,12..13} (5 alike) : Logic  Operator=NOT  AllPortsSameDT=off  OutDataTypeStr=boolean
  Logical Operator{2..5,10..11} (6 alike) : Logic  AllPortsSameDT=off  OutDataTypeStr=boolean
  Logical Operator6 : Logic  Operator=OR  AllPortsSameDT=off  OutDataTypeStr=boolean
  Relational Operator{,1..5,7,9..11} (10 alike) : RelationalOperator  Operator===  OutDataTypeStr=boolean
  Relational Operator13 : RelationalOperator  Operator=<=  OutDataTypeStr=boolean
  Terminator : Terminator
  VJUD_LFCOffRecover_flg : Outport
  wires:
  Logical Operator/1 -> VJUD_LFCOffRecover_flg/1  "VJUD_LFCOffRecover_flg"
  Constant/1 -> Relational Operator/2
  VDINR_EPSLFCStatus_enum/1 -> [VDINR_EPSLFCStatus_enum], Relational Operator/1
  Relational Operator/1 -> Logical Operator3/2
  VDINR_EPSADASAbReason_enum/1 -> Relational Operator1/1, [VDINR_EPSADASAbReason_enum]
  Constant1/1 -> Relational Operator1/2
  Relational Operator1/1 -> Logical Operator3/1
  [VDINR_EPSLFCStatus_enum] -> Relational Operator2/1
  Relational Operator2/1 -> Logical Operator4/2
  Constant2/1 -> Relational Operator3/2
  Relational Operator3/1 -> Logical Operator4/1
  [VDINR_EPSADASAbReason_enum] -> Relational Operator3/1
  Constant3/1 -> Relational Operator2/2
  [VDINR_EPSLFCStatus_enum] -> Relational Operator4/1
  Relational Operator4/1 -> Logical Operator5/2
  Constant4/1 -> Relational Operator5/2
  Relational Operator5/1 -> Logical Operator5/1
  [VDINR_EPSADASAbReason_enum] -> Relational Operator5/1
  Constant5/1 -> Relational Operator4/2
  VDINR_VehSpd_kph/1 -> Relational Operator13/1
  VIFO_InForwardGear_flg/1 -> Logical Operator7/1
  VACC_ACCActing_flg/1 -> Logical Operator1/1
  Constant13/1 -> Add/1
  Constant7/1 -> Add/2
  Add/1 -> Relational Operator13/2
  Logical Operator1/1 -> Logical Operator/1
  Logical Operator7/1 -> Logical Operator/2
  Logical Operator5/1 -> Logical Operator/7
  Logical Operator4/1 -> Logical Operator/6
  Logical Operator3/1 -> Logical Operator/5
  Relational Operator13/1 -> Logical Operator/3
  VIFO_LFCSpdInRange_flg/1 -> Logical Operator8/1
  VFCW_FCWStateHMI_enum/1 -> Relational Operator9/1
  VAEB_AEBStateHMI_enum/1 -> Relational Operator10/1
  Constant12/1 -> Relational Operator9/2
  Constant14/1 -> Relational Operator10/2
  VDINR_LFCOnVCU_flg/1 -> Logical Operator10/1
  VLFC_LFCActing_flg/1 -> Logical Operator10/2
  VIFO_ResidualLaneFinish_flg/1 -> Detect Decrease/1
  VIFO_DegradedFinish_flg/1 -> Detect Decrease1/1
  VIFO_DriverHOD4Disabled_flg/1 -> Logical Operator11/1
  VLFC_LFCState_enum/1 -> Relational Operator7/1, Relational Operator11/1
  Constant10/1 -> Relational Operator11/2
  Relational Operator11/1 -> Logical Operator11/2
  Constant8/1 -> Relational Operator7/2
  Relational Operator7/1 -> Logical Operator2/1
  Logical Operator6/1 -> Logical Operator2/2
  VPER_LeftLaneAvail_flg/1 -> Logical Operator12/1
  VPER_RightLaneAvail_flg/1 -> Logical Operator13/1
  Logical Operator12/1 -> Logical Operator6/1
  Logical Operator13/1 -> Logical Operator6/2
  VIFO_BrakePedalPressed_flg/1 -> Logical Operator/10
  VIFO_DriverShifting_flg/1 -> Logical Operator/9
  VIFO_Curvature4Disable_flg/1 -> Logical Operator/8
  Relational Operator10/1 -> Logical Operator/12
  Relational Operator9/1 -> Logical Operator/11
  VIFO_DriverStrFight_flg/1 -> Logical Operator/13
  Logical Operator10/1 -> Logical Operator/14
  Detect Decrease1/1 -> Logical Operator/16
  Detect Decrease/1 -> Logical Operator/15
  Logical Operator2/1 -> Logical Operator/18
  Logical Operator11/1 -> Logical Operator/17
  VIFO_DriverTurningSignal_flg/1 -> Terminator/1
  ForLCA/1 -> Logical Operator/19
  Logical Operator8/1 -> Logical Operator/4

== system jud/JUD/jud/JLFC/jfc/LFC_ReturnAutoSteering_Conditions ==
  VIFO_LaneNotAvail_flg : Inport
  VIFO_ResidualLaneFinish_flg : Inport  Port=2
  VIFO_DegradedFinish_flg : Inport  Port=3
  Logical Operator : Logic  Inputs=3  AllPortsSameDT=off  OutDataTypeStr=boolean
  Logical Operator1 : Logic  Operator=NOT  Inputs=1  AllPortsSameDT=off  OutDataTypeStr=boolean
  Logical Operator2 : Logic  Operator=NOT  Inputs=1  AllPortsSameDT=off  OutDataTypeStr=boolean
  Logical Operator3 : Logic  Operator=NOT  Inputs=1  AllPortsSameDT=off  OutDataTypeStr=boolean
  VJUD_DegradedToAutoStr_flg : Outport
  wires:
  VIFO_LaneNotAvail_flg/1 -> Logical Operator1/1
  Logical Operator/1 -> VJUD_DegradedToAutoStr_flg/1  "VJUD_DegradedToAutoStr_flg"
  Logical Operator1/1 -> Logical Operator/1
  VIFO_ResidualLaneFinish_flg/1 -> Logical Operator2/1
  VIFO_DegradedFinish_flg/1 -> Logical Operator3/1
  Logical Operator2/1 -> Logical Operator/2
  Logical Operator3/1 -> Logical Operator/3

== system jud/JUD/jud/JLFC/jfc/LFC_SoftenTime_Calculation ==
  KJUD_SoftenTimerThr_s : Constant  Value=KJUD_SoftenTimerThr_s  OutDataTypeStr=single
  VJUD_SoftenTimeThr_s : Outport
  wires:
  KJUD_SoftenTimerThr_s/1 -> VJUD_SoftenTimeThr_s/1  "VJUD_SoftenTimeThr_s"

== system jud/JUD/jud/JLFC/jfc/LFC_Soften_Conditions ==
  VIFO_DriverStrStrong_flg : Inport
  VDINR_EPSLFCStatus_enum : Inport  Port=2
  Constant : Constant  Value=ENUM_EPSLFCSTATUS_TRANSITION
  Logical Operator2 : Logic  Operator=OR  Inputs=1  AllPortsSameDT=off  OutDataTypeStr=boolean
  Relational Operator : RelationalOperator  Operator===  OutDataTypeStr=boolean
  Terminator : Terminator
  VJUD_LFCSoftenReq_flg : Outport
  wires:
  VIFO_DriverStrStrong_flg/1 -> Logical Operator2/1
  Logical Operator2/1 -> VJUD_LFCSoftenReq_flg/1  "VJUD_LFCSoftenReq_flg"
  VDINR_EPSLFCStatus_enum/1 -> Relational Operator/1
  Constant/1 -> Relational Operator/2
  Relational Operator/1 -> Terminator/1

== system jud/JUD/jud/JLFC/jfc/LFC_TempFailureRecover_Conditions ==
  VDINR_EPSLFCStatus_enum : Inport
  VDHP_DisableADASFun_flg : Inport  Port=2
  Constant : Constant  Value=ENUM_EPSLFCSTATUS_OFF
  Constant1 : Constant  Value=ENUM_EPSLFCSTATUS_NOTAVAIL_PERM
  Logical Operator : Logic  Operator=OR  Inputs=3  AllPortsSameDT=off  OutDataTypeStr=boolean
  Logical Operator1 : Logic  Operator=NOT  AllPortsSameDT=off  OutDataTypeStr=boolean
  Relational Operator : RelationalOperator  Operator===  OutDataTypeStr=boolean
  Relational Operator1 : RelationalOperator  Operator===  OutDataTypeStr=boolean
  VJUD_LFCTempFailureRecover_flg : Outport
  wires:
  Logical Operator/1 -> VJUD_LFCTempFailureRecover_flg/1  "VJUD_LFCTempFailureRecover_flg"
  Relational Operator/1 -> Logical Operator/1
  Constant/1 -> Relational Operator/2
  Relational Operator1/1 -> Logical Operator/2
  VDINR_EPSLFCStatus_enum/1 -> Relational Operator1/1, Relational Operator/1
  Constant1/1 -> Relational Operator1/2
  VDHP_DisableADASFun_flg/1 -> Logical Operator1/1
  Logical Operator1/1 -> Logical Operator/3

== system jud/JUD/jud/JLFC/jfc/LFC_Temporary_Conditions ==
  VDINR_EPSLFCStatus_enum : Inport
  VDHP_DisableLFC_flg : Inport  Port=2
  Constant : Constant  Value=ENUM_EPSLFCSTATUS_NOTAVAIL_TEMP
  Logical Operator : Logic  Operator=OR  AllPortsSameDT=off  OutDataTypeStr=boolean
  Relational Operator : RelationalOperator  Operator===  OutDataTypeStr=boolean
  VJUD_LFCTempFailureReq_flg : Outport
  wires:
  Logical Operator/1 -> VJUD_LFCTempFailureReq_flg/1  "VJUD_LFCTempFailureReq_flg"
  VDINR_EPSLFCStatus_enum/1 -> Relational Operator/1
  Constant/1 -> Relational Operator/2
  VDHP_DisableLFC_flg/1 -> Logical Operator/1
  Relational Operator/1 -> Logical Operator/2

== system jud/JUD/jud/JLKA/jka/LKA_CheckNormalFailure_Conditions ==
  VDINR_KeySwitchStatus_enum : Inport
  VDINR_KeySwitchStatusValid_flg : Inport  Port=2
  VDINR_EPSLKAStatus_enum : Inport  Port=3
  VDHP_DisableADASFun_flg : Inport  Port=4
  VIFO_DriverSafetyStatusOk_flg : Inport  Port=5
  VIFO_LatVehicleStatusOk_flg : Inport  Port=6
  VPER_CameraStatus_enum : Inport  Port=7
  Constant : Constant  Value=ENUM_KEYSWITCH_ON
  Constant1 : Constant  Value=ENUM_EPSLFCSTATUS_NOTAVAIL_PERM
  Constant2 : Constant  Value=ENUM_SENSORSTATE_NORMAL
  Logical Operator : Logic  Operator=OR  Inputs=7  AllPortsSameDT=off  OutDataTypeStr=boolean
  Logical Operator2 : Logic  Operator=NOT  AllPortsSameDT=off  OutDataTypeStr=boolean
  Logical Operator3 : Logic  Operator=NOT  AllPortsSameDT=off  OutDataTypeStr=boolean
  Logical Operator4 : Logic  Operator=NOT  AllPortsSameDT=off  OutDataTypeStr=boolean
  Relational Operator : RelationalOperator  Operator=~=  OutDataTypeStr=boolean
  Relational Operator1 : RelationalOperator  Operator===  OutDataTypeStr=boolean
  Relational Operator2 : RelationalOperator  Operator=~=  OutDataTypeStr=boolean
  VJUD_LKACheckNormalFailure_flg : Outport
  wires:
  VDHP_DisableADASFun_flg/1 -> Logical Operator/5
  Constant2/1 -> Relational Operator2/2
  VPER_CameraStatus_enum/1 -> Relational Operator2/1
  VIFO_LatVehicleStatusOk_flg/1 -> Logical Operator4/1
  Constant1/1 -> Relational Operator1/2
  VDINR_EPSLKAStatus_enum/1 -> Relational Operator1/1
  VIFO_DriverSafetyStatusOk_flg/1 -> Logical Operator3/1
  VDINR_KeySwitchStatusValid_flg/1 -> Logical Operator2/1
  Relational Operator/1 -> Logical Operator/1
  Constant/1 -> Relational Operator/2
  VDINR_KeySwitchStatus_enum/1 -> Relational Operator/1
  Logical Operator/1 -> VJUD_LKACheckNormalFailure_flg/1  "VJUD_LKACheckNormalFailure_flg"
  Relational Operator2/1 -> Logical Operator/6
  Relational Operator1/1 -> Logical Operator/7
  Logical Operator2/1 -> Logical Operator/2
  Logical Operator3/1 -> Logical Operator/3
  Logical Operator4/1 -> Logical Operator/4

== system jud/JUD/jud/JLKA/jka/LKA_CheckNormal_Conditions ==
  VDINR_KeySwitchStatus_enum : Inport
  VDINR_KeySwitchStatusValid_flg : Inport  Port=2
  VDINR_EPSLKAStatus_enum : Inport  Port=3
  VDHP_DisableADASFun_flg : Inport  Port=4
  VIFO_DriverSafetyStatusOk_flg : Inport  Port=5
  VIFO_LatVehicleStatusOk_flg : Inport  Port=6
  VPER_CameraStatus_enum : Inport  Port=7
  Constant : Constant  Value=ENUM_KEYSWITCH_ON
  Constant1 : Constant  Value=ENUM_EPSLKASTATUS_OFF
  Constant2 : Constant  Value=ENUM_SENSORSTATE_NORMAL
  Logical Operator : Logic  Inputs=7  AllPortsSameDT=off  OutDataTypeStr=boolean
  Logical Operator1 : Logic  Operator=NOT  AllPortsSameDT=off  OutDataTypeStr=boolean
  Relational Operator : RelationalOperator  Operator===  OutDataTypeStr=boolean
  Relational Operator1 : RelationalOperator  Operator===  OutDataTypeStr=boolean
  Relational Operator2 : RelationalOperator  Operator===  OutDataTypeStr=boolean
  VJUD_LKACheckNormal_flg : Outport
  wires:
  Logical Operator/1 -> VJUD_LKACheckNormal_flg/1  "VJUD_LKACheckNormal_flg"
  VDINR_KeySwitchStatus_enum/1 -> Relational Operator/1
  Constant/1 -> Relational Operator/2
  Relational Operator/1 -> Logical Operator/1
  VDINR_KeySwitchStatusValid_flg/1 -> Logical Operator/2
  VIFO_DriverSafetyStatusOk_flg/1 -> Logical Operator/3
  VDHP_DisableADASFun_flg/1 -> Logical Operator1/1
  VDINR_EPSLKAStatus_enum/1 -> Relational Operator1/1
  Constant1/1 -> Relational Operator1/2
  Relational Operator2/1 -> Logical Operator/5
  VPER_CameraStatus_enum/1 -> Relational Operator2/1
  Constant2/1 -> Relational Operator2/2
  VIFO_LatVehicleStatusOk_flg/1 -> Logical Operator/4
  Relational Operator1/1 -> Logical Operator/6
  Logical Operator1/1 -> Logical Operator/7

== system jud/JUD/jud/JLKA/jka/LKA_Enabled_Conditions ==
  VDINR_LKAEnableH_flg : Inport
  VDINR_LKAEnableHValid_flg : Inport  Port=2
  VDINR_VehSpd_kph : Inport  Port=3
  VIFO_EPSStateChgAllow_flg : Inport  Port=4
  VIFO_InForwardGear_flg : Inport  Port=5
  VLFC_LFCActing_flg : Inport  Port=6
  Constant1 : Constant  Value=KJUD_EPSLimition_kph
  Logical Operator : Logic  Inputs=6  AllPortsSameDT=off  OutDataTypeStr=boolean
  Logical Operator2 : Logic  Operator=NOT  AllPortsSameDT=off  OutDataTypeStr=boolean
  Relational Operator1 : RelationalOperator  OutDataTypeStr=boolean
  Relational Operator7 : RelationalOperator  OutDataTypeStr=boolean
  Timer : hcu_lib/Timer  SystemSampleTime=-1
  VJUD_LFCOffCount4LKAStandby_s : Constant  Value=VJUD_LFCOffCount4LKAStandby_s  OutDataTypeStr=single
  VJUD_LKAEnabledReq_flg : Outport
  wires:
  VDINR_LKAEnableH_flg/1 -> Logical Operator/1
  Logical Operator/1 -> VJUD_LKAEnabledReq_flg/1  "VJUD_LKAEnabledReq_flg"
  VDINR_LKAEnableHValid_flg/1 -> Logical Operator/2
  VDINR_VehSpd_kph/1 -> Relational Operator7/1
  Constant1/1 -> Relational Operator7/2
  VLFC_LFCActing_flg/1 -> Logical Operator2/1
  Relational Operator7/1 -> Logical Operator/3
  VIFO_InForwardGear_flg/1 -> Logical Operator/4
  VIFO_EPSStateChgAllow_flg/1 -> Logical Operator/5
  Logical Operator2/1 -> Timer/Enable
  Relational Operator1/1 -> Logical Operator/6
  Timer/1 -> Relational Operator1/1
  VJUD_LFCOffCount4LKAStandby_s/1 -> Relational Operator1/2

== system jud/JUD/jud/JLKA/jka/LKA_LeftAction_Conditions ==
  VDINR_EPSLKAStatus_enum : Inport
  VIFO_EPSStateChgAllow_flg : Inport  Port=2
  VIFO_TLCLTrigger_flg : Inport  Port=3
  VIFO_TLCRTrigger_flg : Inport  Port=4
  VLKA_LKAActing_flg : Inport  Port=5
  Constant : Constant  Value=ENUM_EPSLKASTATUS_READY
  Logical Operator : Logic  Operator=NOT  AllPortsSameDT=off  OutDataTypeStr=boolean
  Logical Operator3 : Logic  Inputs=5  AllPortsSameDT=off  OutDataTypeStr=boolean
  Logical Operator4 : Logic  Operator=NOT  AllPortsSameDT=off  OutDataTypeStr=boolean
  Relational Operator : RelationalOperator  RequirementInfo={} %GIDa_681efecc_5289_48a6_b694_f7f540d9a041  Operator===  OutDataTypeStr=boolean
  Relational Operator1 : RelationalOperator  OutDataTypeStr=boolean
  Relational Operator2 : RelationalOperator  OutDataTypeStr=boolean
  Timer : hcu_lib/Timer  SystemSampleTime=-1
  Timer1 : hcu_lib/Timer  SystemSampleTime=-1
  VJUD_LKAReActingDelay_s : Constant  Value=VJUD_LKAReActingDelay_s
  VJUD_TLCTriggerReActingDelay_s : Constant  Value=VJUD_TLCTriggerReActingDelay_s
  VJUD_LKALeftActionReq_flg : Outport
  wires:
  Logical Operator3/1 -> VJUD_LKALeftActionReq_flg/1  "VJUD_LKALeftActionReq_flg"
  Constant/1 -> Relational Operator/2
  VDINR_EPSLKAStatus_enum/1 -> Relational Operator/1
  VIFO_TLCRTrigger_flg/1 -> Logical Operator/1
  Timer/1 -> Relational Operator2/1
  VJUD_LKAReActingDelay_s/1 -> Relational Operator2/2
  VIFO_TLCLTrigger_flg/1 -> Logical Operator3/1
  Logical Operator4/1 -> Timer/Enable
  VLKA_LKAActing_flg/1 -> Logical Operator4/1
  VIFO_EPSStateChgAllow_flg/1 -> Logical Operator3/5
  Relational Operator/1 -> Logical Operator3/4
  Relational Operator2/1 -> Logical Operator3/2
  Timer1/1 -> Relational Operator1/1
  VJUD_TLCTriggerReActingDelay_s/1 -> Relational Operator1/2
  Relational Operator1/1 -> Logical Operator3/3
  Logical Operator/1 -> Timer1/Enable
